simulink model "Model_back"  (R2024b)
settings: Solver=FixedStepAuto  StartTime=0.0  StopTime=10  FixedStep=1e-4  RelTol=1e-3
undefined symbols (not defined in the file): param, x0
libraries: slpidlib x1
settings Model: Creator=Nabil  LastModifiedBy=Nabil
settings DebuggingCC: UnderSpecifiedDimensionMsg=warning
settings RTWCC: GenCodeOnly=on

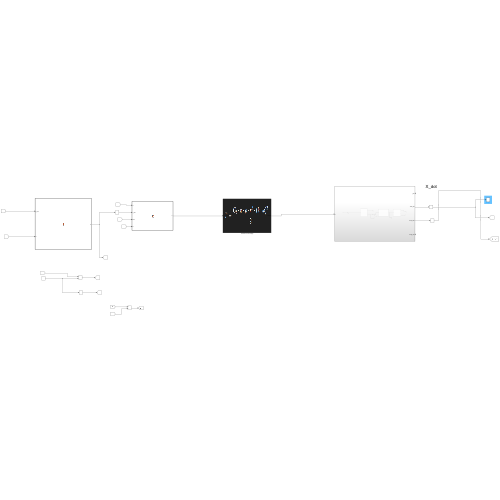
[thumbnail: Simulink's stored preview of the top-level diagram]
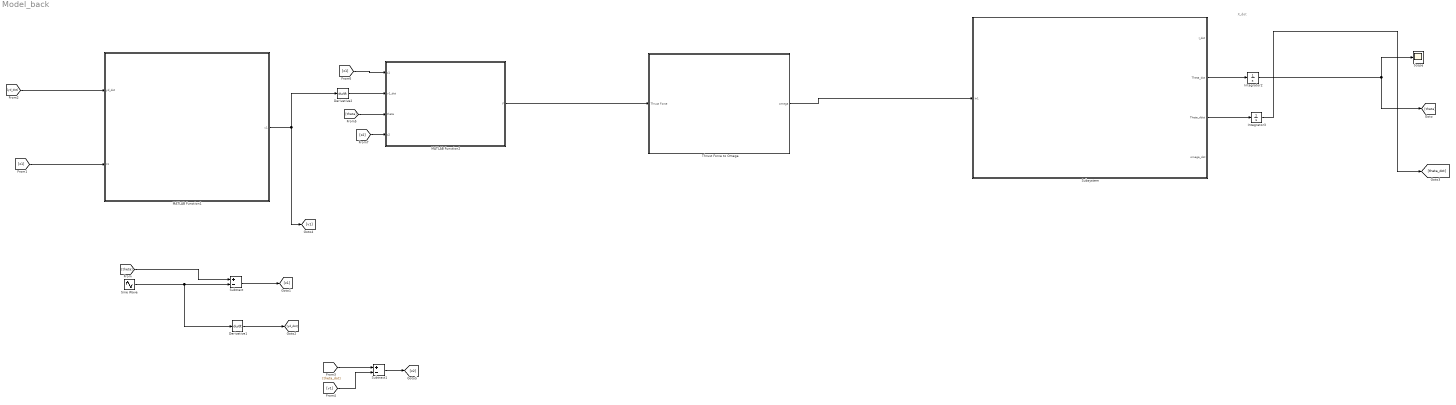
== system Model_back ==
  note: X_dot
  " Thrust Force to Omega" : Subsystem
      mask Display: image('Thrust.png');
  Derivative1 : Derivative
  Derivative2 : Derivative
  Integrator2 : Integrator  InitialCondition=x0(1)
  Integrator3 : Integrator  InitialCondition=x0(2)
  MATLAB Function1 : MATLAB Function  TreatAsAtomicUnit=on
  MATLAB Function2 : MATLAB Function  TreatAsAtomicUnit=on
  Scope : Scope
  Sine Wave : Sin  Amplitude=4  Frequency=5  SampleTime=0
  Subsystem : Subsystem
  Subtract : Sum  Inputs=+-
  Subtract1 : Sum  Inputs=+-
  wires:
  Subsystem/2(Theta_dot) -> Integrator2/1
  Subsystem/3(Theta_ddot) -> Integrator3/1
  Integrator2/1 -> Scope/1, [theta]
  Integrator3/1 -> [theta_dot]
  [theta] -> Subtract/1
  Subtract/1 -> [z1]
  Sine Wave/1 -> Derivative1/1, Subtract/2
  Derivative1/1 -> [yd_dot]
  [yd_dot] -> MATLAB Function1/1(yd_dot)
  [z1] -> MATLAB Function1/2(z1)
  MATLAB Function1/1(v1) -> [v1], Derivative2/1
  [theta_dot] -> Subtract1/1
  [v1] -> Subtract1/2
  Subtract1/1 -> [z2]
  [theta] -> MATLAB Function2/3(theta)
  Derivative2/1 -> MATLAB Function2/2(v1_dot)
  [z1] -> MATLAB Function2/1(z1)
  [z2] -> MATLAB Function2/4(z2)
  " Thrust Force to Omega"/1(omega) -> Subsystem/1(In1)
  MATLAB Function2/1(F) -> " Thrust Force to Omega"/1(Thrust Force)

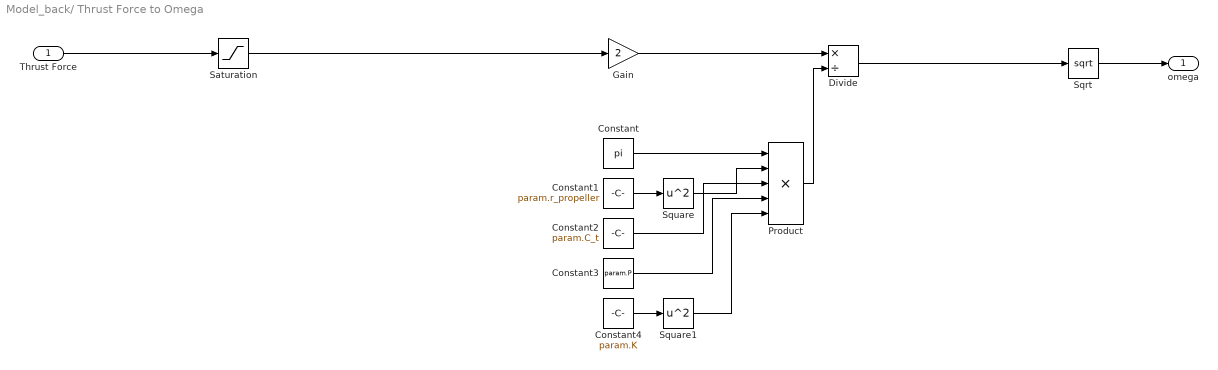
== system Model_back/ Thrust Force to Omega ==
  Thrust Force : Inport
  Constant : Constant  Value=pi
  Constant1 : Constant  Value=param.r_propeller
  Constant2 : Constant  Value=param.C_t
  Constant3 : Constant  Value=param.P
  Constant4 : Constant  Value=param.K
  Divide : Product  Inputs=*/
  Gain : Gain  Gain=2
  Product : Product  Inputs=5
  Saturation : Saturate  UpperLimit=100  LowerLimit=0
  Sqrt : Sqrt
  Square : Math  Operator=square
  Square1 : Math  Operator=square
  omega : Outport
  wires:
  Gain/1 -> Divide/1
  Constant1/1 -> Square/1
  Constant4/1 -> Square1/1
  Square1/1 -> Product/5
  Constant3/1 -> Product/4
  Constant2/1 -> Product/3
  Square/1 -> Product/2
  Constant/1 -> Product/1
  Product/1 -> Divide/2
  Divide/1 -> Sqrt/1
  Sqrt/1 -> omega/1
  Thrust Force/1 -> Saturation/1
  Saturation/1 -> Gain/1

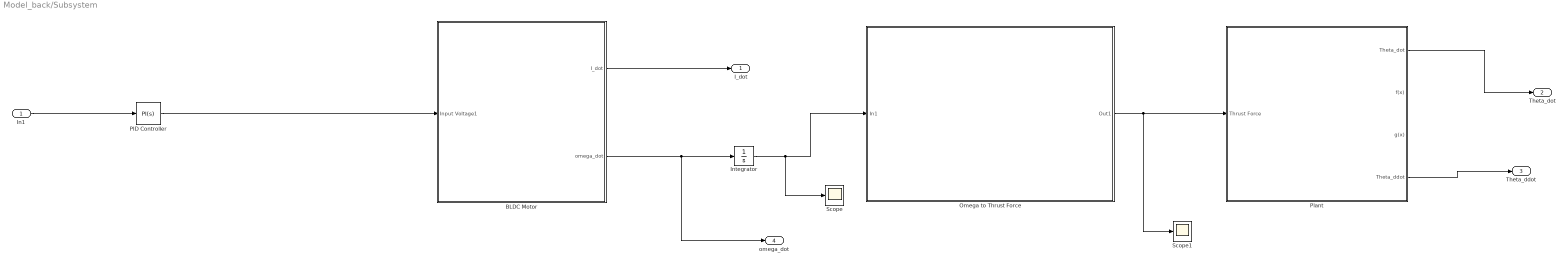
== system Model_back/Subsystem ==
  In1 : Inport
  BLDC Motor : Subsystem
      mask Display: image('2200kv-brushless-motor.jpg');
  Integrator : Integrator
  Omega to Thrust Force : Subsystem
      mask Display: image('Thrust.png');
  PID Controller : slpidlib/PID Controller  Controller=PI  Form=Parallel  TimeDomain=Continuous-time  UseExternalTs=off  SampleTime=-1  IntegratorMethod=Forward Euler  FilterMethod=Forward Euler  ControllerParametersSource=internal  P=0.00672607637527889  I=12.1724881896349  UseKiTs=off  D=0  UseExternalDerivativeSource=off  N=100  UseFilter=on  TunerSelectOption=Transfer Function Based (PID Tuner App)  InitialConditionSource=internal  InitialConditionForIntegrator=0  InitialConditionForFilter=0  DifferentiatorICPrevScaledInput=0  ExternalReset=none  TrackingMode=off  Kt=1  LimitOutput=off  SatLimitsSource=internal  UpperSaturationLimit=inf  LowerSaturationLimit=-inf  LinearizeAsGain=on  AntiWindupMode=none  Kb=1  LimitIntegrator=off  UpperIntegratorSaturationLimit=inf  LowerIntegratorSaturationLimit=-inf  POutMin=[]  POutMax=[]  IOutMin=[]  IOutMax=[]  DOutMin=[]  DOutMax=[]  NOutMin=[]  NOutMax=[]  SumOutMin=[]  SumOutMax=[]  SaturationOutMin=[]  SaturationOutMax=[]  PParamMin=[]  PParamMax=[]  IParamMin=[]  IParamMax=[]  DParamMin=[]  DParamMax=[]  NParamMin=[]  NParamMax=[]  KbParamMin=[]  KbParamMax=[]  KtParamMin=[]  KtParamMax=[]  KbOutMin=[]  KbOutMax=[]  KtOutMin=[]  KtOutMax=[]  IntegratorOutMin=[]  IntegratorOutMax=[]  FilterOutMin=[]  FilterOutMax=[]  SumI1OutMin=[]  SumI1OutMax=[]  SumI2OutMin=[]  SumI2OutMax=[]  SumI3OutMin=[]  SumI3OutMax=[]  SumI4OutMin=[]  SumI4OutMax=[]  SumDOutMin=[]  SumDOutMax=[]  DifferentiatorOutMin=[]  DifferentiatorOutMax=[]  FilterDiffOutCoefMin=[]  FilterDiffOutCoefMax=[]  ReciprocalOutMin=[]  ReciprocalOutMax=[]  SumDenOutMin=[]  SumDenOutMax=[]  SumNumOutMin=[]  SumNumOutMax=[]  DivideOutMin=[]  DivideOutMax=[]  UdiffTsProdOutMin=[]  UdiffTsProdOutMax=[]  NTsProdOutMin=[]  NTsProdOutMax=[]  UintegralTsProdOutMin=[]  UintegralTsProdOutMax=[]  UngainTsProdOutMin=[]  UngainTsProdOutMax=[]  ClampingZeroOutDataTypeStr=Inherit: Inherit via back propagation  ClampingZeroOutMin=[]  ClampingZeroOutMax=[]  FilterDenConstantOutDataTypeStr=Inherit: Inherit via back propagation  FilterDenConstantOutMin=[]  FilterDenConstantOutMax=[]  PCopyOutDataTypeStr=Inherit: Inherit via back propagation  PCopyOutMin=[]  PCopyOutMax=[]  NCopyOutDataTypeStr=Inherit: Inherit via back propagation  NCopyOutMin=[]  NCopyOutMax=[]  IntegratorContinuousStateAttributes=''  IntegratorStateMustResolveToSignalObject=off  IntegratorRTWStateStorageClass=Auto  FilterContinuousStateAttributes=''  FilterStateMustResolveToSignalObject=off  FilterRTWStateStorageClass=Auto  ParallelPVariant=InternalParameters  IdealPVariant=Disabled  IVariant=InternalParameters  DVariant=Disabled  IntegratorVariant=Continuous  SatVariant=Disabled  AWVariant=Passthrough  PCopyVariant=Disabled  TRVariant=Disabled  FdbkBlocksVariant=Forward  IdealPFdbkVariant=Disabled  SatFdbkVariant=Disabled  DerivativeFilterVariant=Disabled  NVariant=Disabled  NCopyVariant=Disabled_SignalSpec  FilterICVariant=Disabled  IntegratorICVariant=InternalICs  ExternalResetVariant=Disabled  TRSumVariant=Passthrough  SumFdbkVariant=Disabled  SumVariant=Sum_PI  TsampFilterVariant=InternalTs  TsampNgainVariant=Passthrough  TsampIntegralVariant=Disabled_SignalSpec  ExternalSaturationOutDataTypeStr=Inherit: Same as second input  DerivativeSourceVariant=Disabled  PreIntVariant=InternalPreInt
  Plant : Subsystem
      mask Display: image('1DoF.png');
  Scope : Scope
  Scope1 : Scope
  I_dot : Outport
  Theta_dot : Outport  Port=2
  Theta_ddot : Outport  Port=3
  omega_dot : Outport  Port=4
  wires:
  BLDC Motor/1(I_dot) -> I_dot/1
  BLDC Motor/2(omega_dot) -> omega_dot/1, Integrator/1
  Integrator/1 -> Scope/1, Omega to Thrust Force/1(In1)
  Omega to Thrust Force/1(Out1) -> Scope1/1, Plant/1(Thrust Force)
  Plant/4(Theta_ddot) -> Theta_ddot/1
  Plant/1(Theta_dot) -> Theta_dot/1
  PID Controller/1 -> BLDC Motor/1(Input Voltage1)
  In1/1 -> PID Controller/1

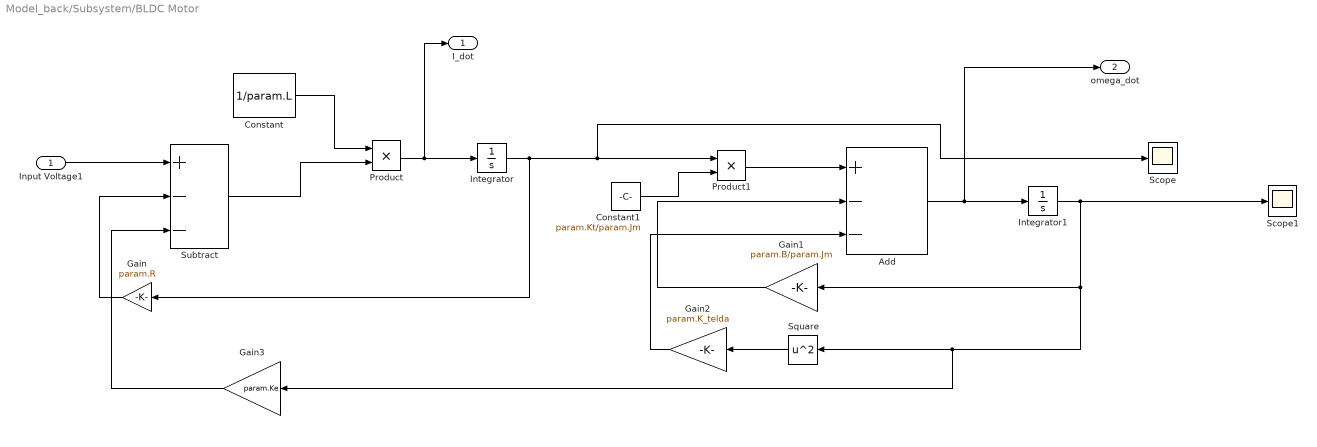
== system Model_back/Subsystem/BLDC Motor ==
  Input Voltage1 : Inport
  Add : Sum  Inputs=+--
  Constant : Constant  Value=1/param.L
  Constant1 : Constant  Value=param.Kt/param.Jm
  Gain : Gain  Gain=param.R
  Gain1 : Gain  Gain=param.B/param.Jm
  Gain2 : Gain  Gain=param.K_telda
  Gain3 : Gain  Gain=param.Ke
  Integrator : Integrator  InitialCondition=x0(4)
  Integrator1 : Integrator  InitialCondition=x0(3)
  Product : Product
  Product1 : Product
  Scope : Scope
  Scope1 : Scope
  Square : Math  Operator=square
  Subtract : Sum  Inputs=+--
  I_dot : Outport
  omega_dot : Outport  Port=2
  wires:
  Constant/1 -> Product/1
  Input Voltage1/1 -> Subtract/1
  Product/1 -> I_dot/1, Integrator/1
  Integrator/1 -> Gain/1, Scope/1, Product1/1
  Gain/1 -> Subtract/2
  Subtract/1 -> Product/2
  Constant1/1 -> Product1/2
  Product1/1 -> Add/1
  Add/1 -> omega_dot/1, Integrator1/1
  Square/1 -> Gain2/1
  Gain2/1 -> Add/3
  Gain1/1 -> Add/2
  Integrator1/1 -> Gain3/1, Square/1, Gain1/1, Scope1/1
  Gain3/1 -> Subtract/3

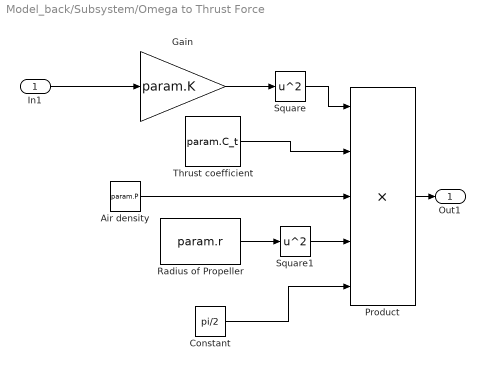
== system Model_back/Subsystem/Omega to Thrust Force ==
  In1 : Inport
  Air density : Constant  Value=param.P
  Constant : Constant  Value=pi/2
  Gain : Gain  Gain=param.K
  Product : Product  Inputs=5
  Radius of Propeller : Constant  Value=param.r
  Square : Math  Operator=square
  Square1 : Math  Operator=square
  Thrust coefficient : Constant  Value=param.C_t
  Out1 : Outport
  wires:
  In1/1 -> Gain/1
  Air density/1 -> Product/3
  Constant/1 -> Product/5
  Thrust coefficient/1 -> Product/2
  Square/1 -> Product/1
  Square1/1 -> Product/4
  Radius of Propeller/1 -> Square1/1
  Gain/1 -> Square/1
  Product/1 -> Out1/1

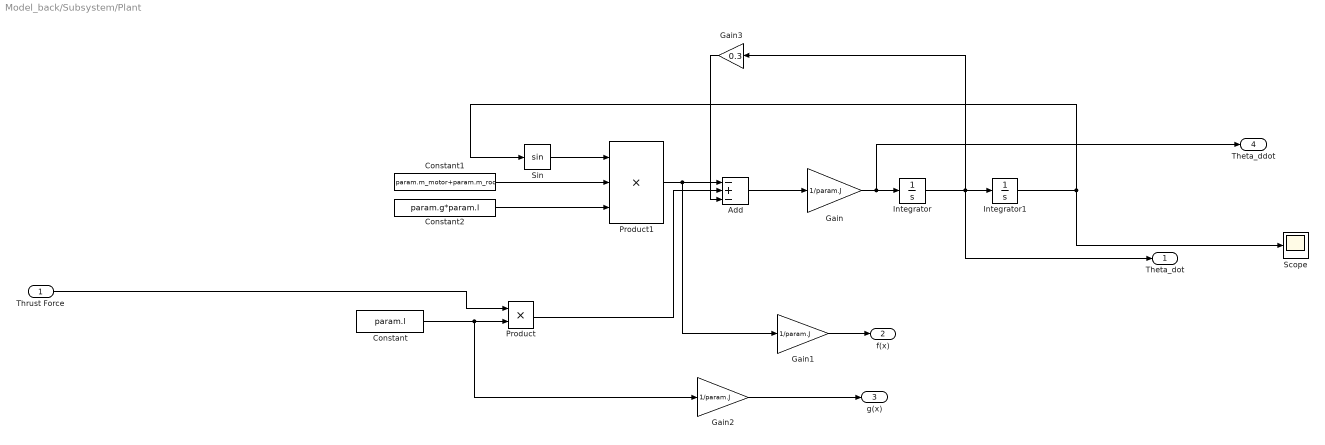
== system Model_back/Subsystem/Plant ==
  Thrust Force : Inport
  Add : Sum  Inputs=-+-
  Constant : Constant  Value=param.l
  Constant1 : Constant  Value=param.m_motor+param.m_rod
  Constant2 : Constant  Value=param.g*param.l
  Gain : Gain  Gain=1/param.J
  Gain1 : Gain  Gain=1/param.J
  Gain2 : Gain  Gain=1/param.J
  Gain3 : Gain  Gain=0.3
  Integrator : Integrator  InitialCondition=x0(2)
  Integrator1 : Integrator  InitialCondition=x0(1)
  Product : Product
  Product1 : Product  Inputs=3
  Scope : Scope
  Sin : Trigonometry
  Theta_dot : Outport
  f(x) : Outport  Port=2
  g(x) : Outport  Port=3
  Theta_ddot : Outport  Port=4
  wires:
  Integrator1/1 -> Sin/1, Scope/1
  Constant/1 -> Gain2/1, Product/2
  Gain/1 -> Theta_ddot/1, Integrator/1
  Integrator/1 -> Gain3/1, Theta_dot/1, Integrator1/1
  Sin/1 -> Product1/1
  Product1/1 -> Gain1/1, Add/1
  Add/1 -> Gain/1
  Constant1/1 -> Product1/2
  Constant2/1 -> Product1/3
  Product/1 -> Add/2
  Thrust Force/1 -> Product/1
  Gain1/1 -> f(x)/1
  Gain2/1 -> g(x)/1
  Gain3/1 -> Add/3

== matlab function Model_back/MATLAB Function1 ==
  data: yd_dot input; v1 output; z1 input
function v1 = fcn(yd_dot,z1)


k1 = 10;
v1 = yd_dot - k1*z1;

== matlab function Model_back/MATLAB Function2 ==
  data: z1 input; F output; v1_dot input; theta input; z2 input
function F = fcn(z1,v1_dot,theta,z2)

k2 =10;

F = 0.06133*(-z1 + v1_dot + 40*sin(theta) -k2*z2);
